simulink library "LiBatteryElements_lib"  (R2020b)
settings: Solver=VariableStepAuto  StartTime=0.0  StopTime=10.0  RelTol=1e-3
values from neighbouring files (symbols this model uses):
  A_an = 2.5e13    (= 25000000000000)    [main_cell.m]
  A_ca = 2.55e14    (= 255000000000000)    [main_cell.m]
  A_sei = 2.25e15    (= 2.25e+15)    [main_cell.m]
  capacity = 4.5    [Cell_1_RC_25.mat]    (also in Cell_43_RC_25.mat; parameters.mat = 10)
  E_an = 2.24e-19    [main_cell.m]
  E_ca = 2.64e-19    [main_cell.m]
  E_sei = 2.24e-19    [main_cell.m]
  h_an = 1714*1000    (= 1714000)    [main_cell.m]
  h_ca = 790*1000    (= 790000)    [main_cell.m]
  h_sei = 257*1000    (= 257000)    [main_cell.m]
  k_b = 1.3806e-23    [main_cell.m]
  m_an = 19.107/1000    (= 0.019107)    [main_cell.m]
  m_ca = 36.56/1000    (= 0.03656)    [main_cell.m]
  x_an_0 = 0.75    [main_cell.m]
  x_sei_0 = 0.15    [main_cell.m]
  z_0 = 0.033    [main_cell.m]
undefined symbols (not defined in the file or in its folder): gcbh, simscape, T_init
libraries: fl_lib x14, $bdroot x4, nesl_utility x4
settings Model: Creator=Vivian  LastModifiedBy=Vivian

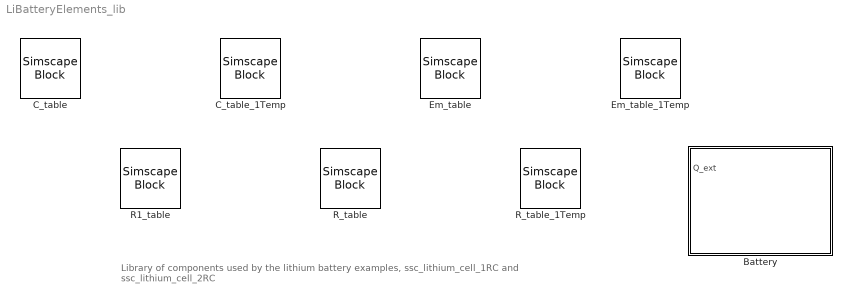
== system LiBatteryElements_lib ==
  note: Library of components used by the lithium battery examples, ssc_lithium_cell_1RC and ssc_lithium_cell_2RC
  Battery : Subsystem
  C_table : SimscapeBlock  DialogController=NetworkEngine.DynNeDlgSource  LoadFcn=simscape.compiler.sli.internal.callback('LoadFcn',gcbh);  SourceFile=LiBatteryElements.C_table  mask(C_table){ComponentPath=LiBatteryElements.C_table, ComponentVariants=["LiBatteryElements.C_table"], ComponentVariantNames=["C_table"], ClassName=C_table, SchemaVersion=1, C_Table=ones(5, 3), C_Table_unit=F, C_Table_conf=compiletime, SOC_Table=[0; .1; .5; .9; 1], SOC_Table_unit=1, SOC_Table_conf=compiletime, Temp_Table=[273.15, 293.15, 313.15], Temp_Table_unit=K, Temp_Table_conf=compiletime, v0=0, v0_unit=V, v0_conf=compiletime}
      mask prompts: C_Table "Matrix of capacitance values, C(SOC,T)"; SOC_Table "State of charge (SOC) breakpoints"; Temp_Table "Temperature (T) breakpoints"; v0 "Initial voltage across capacitor"
      mask help: Models a capacitor where the capacitance value (C) depends on an external physical signal inputs SOC and T. It is assumed that the capacitance value is slowly varying with time, and hence the equation i = C*dv/dt holds.
      mask init:
      | simscape.compiler.sli.internal.preinitmask(gcb);
      settings: CopyFcn=simscape.compiler.sli.internal.callback('CopyFcn',gcbh);  DeleteFcn=simscape.compiler.sli.internal.callback('DeleteFcn',gcbh);  ModelCloseFcn=simscape.compiler.sli.internal.callback('ModelCloseFcn',gcbh);  PreSaveFcn=simscape.compiler.sli.internal.callback('PreSaveFcn',gcbh);  PostSaveFcn=simscape.compiler.sli.internal.callback('PostSaveFcn',gcbh);  PreCopyFcn=simscape.compiler.sli.internal.callback('PreCopyFcn',gcbh);  PreDeleteFcn=simscape.compiler.sli.internal.callback('PreDeleteFcn',gcbh);  InternalSimscapePortConfiguration="{\"Bottom\":[],\"Left\":[{\"id\":\"p\",\"label\":\"+\",\"type\":\"foundation.electrical.electrical\"},{\"id\":\"T\",\"label\":\"T\",\"type\":\"input\"},{\"id\":\"SOC\",\"label\":\"SOC\",\"type\":\"input\"}],\"Right\":[{\"id\":\"n\",\"label\":\"-\",\"type\":\"foundation.electrical.electrical\"}],\"Top\":[]}"
      mask Help: web(nesl_help(gcbh))
      mask TypeOptions C_Table_unit: F | pF | nF | uF | mF
      mask TypeOptions C_Table_conf: compiletime | runtime
      mask TypeOptions SOC_Table_unit: 1
      mask TypeOptions SOC_Table_conf: compiletime | runtime
      mask TypeOptions Temp_Table_unit: K | degC | degF | degR | deltaK | deltadegC | deltadegF | deltadegR
      mask TypeOptions Temp_Table_conf: compiletime | runtime
      mask TypeOptions v0_unit: V | mV | kV
      mask TypeOptions v0_conf: compiletime | runtime
  C_table_1Temp : SimscapeBlock  DialogController=NetworkEngine.DynNeDlgSource  LoadFcn=simscape.compiler.sli.internal.callback('LoadFcn',gcbh);  SourceFile=LiBatteryElements.C_table_1Temp  mask(C_table_1Temp){ComponentPath=LiBatteryElements.C_table_1Temp, ComponentVariants=["LiBatteryElements.C_table_1Temp"], ComponentVariantNames=["C_table_1Temp"], ClassName=C_table_1Temp, SchemaVersion=1, C_Table=ones(5, 1), C_Table_unit=F, C_Table_conf=compiletime, SOC_Table=[0; .1; .5; .9; 1], SOC_Table_unit=1, SOC_Table_conf=compiletime, v0=0, v0_unit=V, v0_conf=compiletime}
      mask prompts: C_Table "Vector of capacitance values"; SOC_Table "Corresponding SOC breakpoints"; v0 "Initial voltage across capacitor"
      mask help: Models a capacitor where the capacitance value (C) depends on an external physical signal input SOC. It is assumed that the capacitance value is slowly varying with time, and hence the equation i = C*dv/dt holds.
      mask init:
      | simscape.compiler.sli.internal.preinitmask(gcb);
      settings: CopyFcn=simscape.compiler.sli.internal.callback('CopyFcn',gcbh);  DeleteFcn=simscape.compiler.sli.internal.callback('DeleteFcn',gcbh);  ModelCloseFcn=simscape.compiler.sli.internal.callback('ModelCloseFcn',gcbh);  PreSaveFcn=simscape.compiler.sli.internal.callback('PreSaveFcn',gcbh);  PostSaveFcn=simscape.compiler.sli.internal.callback('PostSaveFcn',gcbh);  PreCopyFcn=simscape.compiler.sli.internal.callback('PreCopyFcn',gcbh);  PreDeleteFcn=simscape.compiler.sli.internal.callback('PreDeleteFcn',gcbh);  InternalSimscapePortConfiguration="{\"Bottom\":[],\"Left\":[{\"id\":\"p\",\"label\":\"+\",\"type\":\"foundation.electrical.electrical\"},{\"id\":\"SOC\",\"label\":\"SOC\",\"type\":\"input\"}],\"Right\":[{\"id\":\"n\",\"label\":\"-\",\"type\":\"foundation.electrical.electrical\"}],\"Top\":[]}"
      mask Help: web(nesl_help(gcbh))
      mask TypeOptions C_Table_unit: F | pF | nF | uF | mF
      mask TypeOptions C_Table_conf: compiletime | runtime
      mask TypeOptions SOC_Table_unit: 1
      mask TypeOptions SOC_Table_conf: compiletime | runtime
      mask TypeOptions v0_unit: V | mV | kV
      mask TypeOptions v0_conf: compiletime | runtime
  Em_table : SimscapeBlock  DialogController=NetworkEngine.DynNeDlgSource  LoadFcn=simscape.compiler.sli.internal.callback('LoadFcn',gcbh);  SourceFile=LiBatteryElements.Em_table  mask(Em_table){ComponentPath=LiBatteryElements.Em_table, ComponentVariants=["LiBatteryElements.Em_table"], ComponentVariantNames=["Em_table"], ClassName=Em_table, SchemaVersion=1, C_Table=[29, 30, 31], C_Table_unit=hr*A, C_Table_conf=compiletime, Em_Table=3.8 * ones(5, 3), Em_Table_unit=V, Em_Table_conf=compiletime, SOC_Table=[0; .1; .5; .9; 1], SOC_Table_unit=1, SOC_Table_conf=compiletime, Temp_Table=[273.15, 293.15, 313.15], Temp_Table_unit=K, Temp_Table_conf=compiletime, Qinit=0, Qinit_unit=hr*A, Qinit_conf=compiletime}
      mask prompts: C_Table "Capacity values at specified temperature breakpoints"; Em_Table "Matrix of voltage values, Em(SOC,T)"; SOC_Table "State of charge (SOC) breakpoints"; Temp_Table "Temperature (T) breakpoints"; Qinit "Initial charge deficit"
      mask help: This block implements the cell's main branch voltage source, and determines values for capacity (C) and state of charge (SOC). The defining equations depend on cell temperature, T.
      mask init:
      | simscape.compiler.sli.internal.preinitmask(gcb);
      settings: CopyFcn=simscape.compiler.sli.internal.callback('CopyFcn',gcbh);  DeleteFcn=simscape.compiler.sli.internal.callback('DeleteFcn',gcbh);  ModelCloseFcn=simscape.compiler.sli.internal.callback('ModelCloseFcn',gcbh);  PreSaveFcn=simscape.compiler.sli.internal.callback('PreSaveFcn',gcbh);  PostSaveFcn=simscape.compiler.sli.internal.callback('PostSaveFcn',gcbh);  PreCopyFcn=simscape.compiler.sli.internal.callback('PreCopyFcn',gcbh);  PreDeleteFcn=simscape.compiler.sli.internal.callback('PreDeleteFcn',gcbh);  InternalSimscapePortConfiguration="{\"Bottom\":[],\"Left\":[{\"id\":\"p\",\"label\":\"+\",\"type\":\"foundation.electrical.electrical\"},{\"id\":\"C\",\"label\":\"C\",\"type\":\"output\"},{\"id\":\"SOC\",\"label\":\"SOC\",\"type\":\"output\"}],\"Right\":[{\"id\":\"n\",\"label\":\"-\",\"type\":\"foundation.electrical.electrical\"},{\"id\":\"T\",\"label\":\"T\",\"type\":\"input\"}],\"Top\":[]}"
      mask Help: web(nesl_help(gcbh))
      mask TypeOptions C_Table_unit: C | hr*A
      mask TypeOptions C_Table_conf: compiletime | runtime
      mask TypeOptions Em_Table_unit: V | mV | kV
      mask TypeOptions Em_Table_conf: compiletime | runtime
      mask TypeOptions SOC_Table_unit: 1
      mask TypeOptions SOC_Table_conf: compiletime | runtime
      mask TypeOptions Temp_Table_unit: K | degC | degF | degR | deltaK | deltadegC | deltadegF | deltadegR
      mask TypeOptions Temp_Table_conf: compiletime | runtime
      mask TypeOptions Qinit_unit: C | hr*A
      mask TypeOptions Qinit_conf: compiletime | runtime
  Em_table_1Temp : SimscapeBlock  DialogController=NetworkEngine.DynNeDlgSource  LoadFcn=simscape.compiler.sli.internal.callback('LoadFcn',gcbh);  SourceFile=LiBatteryElements.Em_table_1Temp  mask(Em_table_1Temp){ComponentPath=LiBatteryElements.Em_table_1Temp, ComponentVariants=["LiBatteryElements.Em_table_1Temp"], ComponentVariantNames=["Em_table_1Temp"], ClassName=Em_table_1Temp, SchemaVersion=1, Em_Table=3.8 * ones(5, 1), Em_Table_unit=V, Em_Table_conf=compiletime, SOC_Table=[0; .1; .5; .9; 1], SOC_Table_unit=1, SOC_Table_conf=compiletime, C=30, C_unit=hr*A, C_conf=compiletime, Qinit=0, Qinit_unit=hr*A, Qinit_conf=compiletime}
      mask prompts: Em_Table "Vector of voltage values, Em"; SOC_Table "Corresponding SOC breakpoints"; C "Capacity (scalar)"; Qinit "Initial charge deficit"
      mask help: This block implements the main branch voltage source, capacity, and state of charge (SOC). The defining equations are assumed not to depend on temperature.
      mask init:
      | simscape.compiler.sli.internal.preinitmask(gcb);
      settings: CopyFcn=simscape.compiler.sli.internal.callback('CopyFcn',gcbh);  DeleteFcn=simscape.compiler.sli.internal.callback('DeleteFcn',gcbh);  ModelCloseFcn=simscape.compiler.sli.internal.callback('ModelCloseFcn',gcbh);  PreSaveFcn=simscape.compiler.sli.internal.callback('PreSaveFcn',gcbh);  PostSaveFcn=simscape.compiler.sli.internal.callback('PostSaveFcn',gcbh);  PreCopyFcn=simscape.compiler.sli.internal.callback('PreCopyFcn',gcbh);  PreDeleteFcn=simscape.compiler.sli.internal.callback('PreDeleteFcn',gcbh);  InternalSimscapePortConfiguration="{\"Bottom\":[],\"Left\":[{\"id\":\"p\",\"label\":\"+\",\"type\":\"foundation.electrical.electrical\"},{\"id\":\"SOC\",\"label\":\"SOC\",\"type\":\"output\"}],\"Right\":[{\"id\":\"n\",\"label\":\"-\",\"type\":\"foundation.electrical.electrical\"}],\"Top\":[]}"
      mask Help: web(nesl_help(gcbh))
      mask TypeOptions Em_Table_unit: V | mV | kV
      mask TypeOptions Em_Table_conf: compiletime | runtime
      mask TypeOptions SOC_Table_unit: 1
      mask TypeOptions SOC_Table_conf: compiletime | runtime
      mask TypeOptions C_unit: C | hr*A
      mask TypeOptions C_conf: compiletime | runtime
      mask TypeOptions Qinit_unit: C | hr*A
      mask TypeOptions Qinit_conf: compiletime | runtime
  R1_table : SimscapeBlock  DialogController=NetworkEngine.DynNeDlgSource  LoadFcn=simscape.compiler.sli.internal.callback('LoadFcn',gcbh);  SourceFile=LiBatteryElements.R1_table  mask(R1_table){ComponentPath=LiBatteryElements.R1_table, ComponentVariants=["LiBatteryElements.R1_table"], ComponentVariantNames=["R1_table"], ClassName=R1_table, SchemaVersion=1, R_Table=1e-3 * ones(5, 3), R_Table_unit=Ohm, R_Table_conf=compiletime, SOC_Table=[0; .1; .5; .9; 1], SOC_Table_unit=1, SOC_Table_conf=compiletime, Temp_Table=[273.15, 293.15, 313.15], Temp_Table_unit=K, Temp_Table_conf=compiletime}
      mask prompts: R_Table "Matrix of resistance values, R(SOC,T)"; SOC_Table "State of charge (SOC) breakpoints"; Temp_Table "Temperature (T) breakpoints"
      mask help: Models a resistor where the resistance value (R) depends on an external physical signal inputs SOC and T.
      mask init:
      | simscape.compiler.sli.internal.preinitmask(gcb);
      settings: CopyFcn=simscape.compiler.sli.internal.callback('CopyFcn',gcbh);  DeleteFcn=simscape.compiler.sli.internal.callback('DeleteFcn',gcbh);  ModelCloseFcn=simscape.compiler.sli.internal.callback('ModelCloseFcn',gcbh);  PreSaveFcn=simscape.compiler.sli.internal.callback('PreSaveFcn',gcbh);  PostSaveFcn=simscape.compiler.sli.internal.callback('PostSaveFcn',gcbh);  PreCopyFcn=simscape.compiler.sli.internal.callback('PreCopyFcn',gcbh);  PreDeleteFcn=simscape.compiler.sli.internal.callback('PreDeleteFcn',gcbh);  InternalSimscapePortConfiguration="{\"Bottom\":[],\"Left\":[{\"id\":\"p\",\"label\":\"+\",\"type\":\"foundation.electrical.electrical\"},{\"id\":\"T\",\"label\":\"T\",\"type\":\"input\"},{\"id\":\"SOC\",\"label\":\"SOC\",\"type\":\"input\"}],\"Right\":[{\"id\":\"n\",\"label\":\"-\",\"type\":\"foundation.electrical.electrical\"},{\"id\":\"pow\",\"label\":\"POW\",\"type\":\"output\"}],\"Top\":[]}"
      mask Help: web(nesl_help(gcbh))
      mask TypeOptions R_Table_unit: Ohm | kOhm | MOhm | GOhm
      mask TypeOptions R_Table_conf: compiletime | runtime
      mask TypeOptions SOC_Table_unit: 1
      mask TypeOptions SOC_Table_conf: compiletime | runtime
      mask TypeOptions Temp_Table_unit: K | degC | degF | degR | deltaK | deltadegC | deltadegF | deltadegR
      mask TypeOptions Temp_Table_conf: compiletime | runtime
  R_table : SimscapeBlock  DialogController=NetworkEngine.DynNeDlgSource  LoadFcn=simscape.compiler.sli.internal.callback('LoadFcn',gcbh);  SourceFile=LiBatteryElements.R_table  mask(R_table){ComponentPath=LiBatteryElements.R_table, ComponentVariants=["LiBatteryElements.R_table"], ComponentVariantNames=["R_table"], ClassName=R_table, SchemaVersion=1, R_Table=1e-3 * ones(5, 3), R_Table_unit=Ohm, R_Table_conf=compiletime, SOC_Table=[0; .1; .5; .9; 1], SOC_Table_unit=1, SOC_Table_conf=compiletime, Temp_Table=[273.15, 293.15, 313.15], Temp_Table_unit=K, Temp_Table_conf=compiletime}
      mask prompts: R_Table "Matrix of resistance values, R(SOC,T)"; SOC_Table "State of charge (SOC) breakpoints"; Temp_Table "Temperature (T) breakpoints"
      mask help: Models a resistor where the resistance value (R) depends on an external physical signal inputs SOC and T.
      mask init:
      | simscape.compiler.sli.internal.preinitmask(gcb);
      settings: CopyFcn=simscape.compiler.sli.internal.callback('CopyFcn',gcbh);  DeleteFcn=simscape.compiler.sli.internal.callback('DeleteFcn',gcbh);  ModelCloseFcn=simscape.compiler.sli.internal.callback('ModelCloseFcn',gcbh);  PreSaveFcn=simscape.compiler.sli.internal.callback('PreSaveFcn',gcbh);  PostSaveFcn=simscape.compiler.sli.internal.callback('PostSaveFcn',gcbh);  PreCopyFcn=simscape.compiler.sli.internal.callback('PreCopyFcn',gcbh);  PreDeleteFcn=simscape.compiler.sli.internal.callback('PreDeleteFcn',gcbh);  InternalSimscapePortConfiguration="{\"Bottom\":[],\"Left\":[{\"id\":\"p\",\"label\":\"+\",\"type\":\"foundation.electrical.electrical\"},{\"id\":\"T\",\"label\":\"T\",\"type\":\"input\"},{\"id\":\"SOC\",\"label\":\"SOC\",\"type\":\"input\"}],\"Right\":[{\"id\":\"n\",\"label\":\"-\",\"type\":\"foundation.electrical.electrical\"},{\"id\":\"pow\",\"label\":\"POW\",\"type\":\"output\"}],\"Top\":[]}"
      mask Help: web(nesl_help(gcbh))
      mask TypeOptions R_Table_unit: Ohm | kOhm | MOhm | GOhm
      mask TypeOptions R_Table_conf: compiletime | runtime
      mask TypeOptions SOC_Table_unit: 1
      mask TypeOptions SOC_Table_conf: compiletime | runtime
      mask TypeOptions Temp_Table_unit: K | degC | degF | degR | deltaK | deltadegC | deltadegF | deltadegR
      mask TypeOptions Temp_Table_conf: compiletime | runtime
  R_table_1Temp : SimscapeBlock  DialogController=NetworkEngine.DynNeDlgSource  LoadFcn=simscape.compiler.sli.internal.callback('LoadFcn',gcbh);  SourceFile=LiBatteryElements.R_table_1Temp  mask(R_table_1Temp){ComponentPath=LiBatteryElements.R_table_1Temp, ComponentVariants=["LiBatteryElements.R_table_1Temp"], ComponentVariantNames=["R_table_1Temp"], ClassName=R_table_1Temp, SchemaVersion=1, R_Table=1e-3 * ones(5, 1), R_Table_unit=Ohm, R_Table_conf=compiletime, SOC_Table=[0; .1; .5; .9; 1], SOC_Table_unit=1, SOC_Table_conf=compiletime}
      mask prompts: R_Table "Vector of resistance values"; SOC_Table "Corresponding SOC breakpoints"
      mask help: Models a resistor where the resistance value (R) depends on an external physical signal input SOC.
      mask init:
      | simscape.compiler.sli.internal.preinitmask(gcb);
      settings: CopyFcn=simscape.compiler.sli.internal.callback('CopyFcn',gcbh);  DeleteFcn=simscape.compiler.sli.internal.callback('DeleteFcn',gcbh);  ModelCloseFcn=simscape.compiler.sli.internal.callback('ModelCloseFcn',gcbh);  PreSaveFcn=simscape.compiler.sli.internal.callback('PreSaveFcn',gcbh);  PostSaveFcn=simscape.compiler.sli.internal.callback('PostSaveFcn',gcbh);  PreCopyFcn=simscape.compiler.sli.internal.callback('PreCopyFcn',gcbh);  PreDeleteFcn=simscape.compiler.sli.internal.callback('PreDeleteFcn',gcbh);  InternalSimscapePortConfiguration="{\"Bottom\":[],\"Left\":[{\"id\":\"p\",\"label\":\"+\",\"type\":\"foundation.electrical.electrical\"},{\"id\":\"SOC\",\"label\":\"SOC\",\"type\":\"input\"}],\"Right\":[{\"id\":\"n\",\"label\":\"-\",\"type\":\"foundation.electrical.electrical\"}],\"Top\":[]}"
      mask Help: web(nesl_help(gcbh))
      mask TypeOptions R_Table_unit: Ohm | kOhm | MOhm | GOhm
      mask TypeOptions R_Table_conf: compiletime | runtime
      mask TypeOptions SOC_Table_unit: 1
      mask TypeOptions SOC_Table_conf: compiletime | runtime

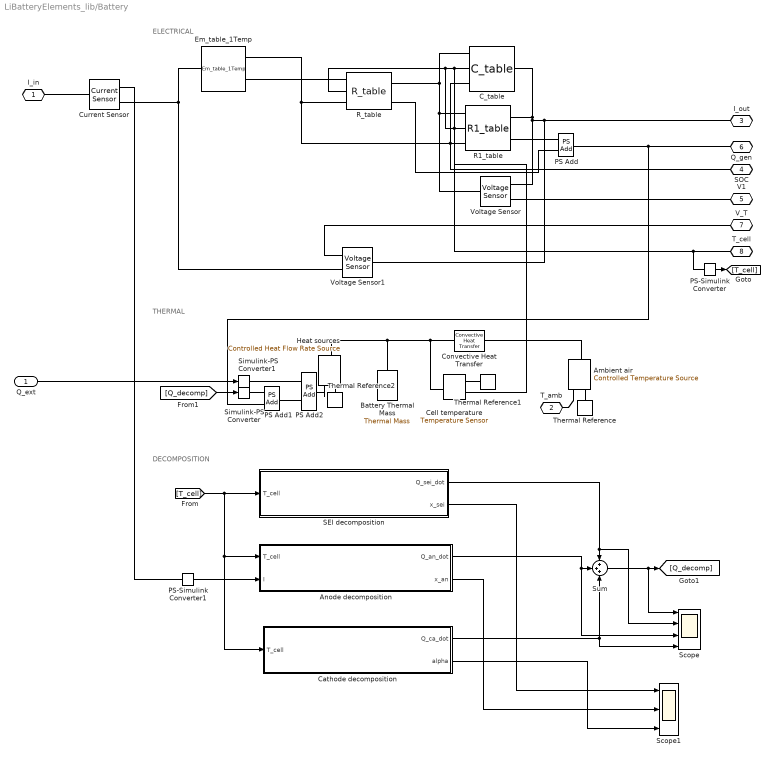
== system LiBatteryElements_lib/Battery ==
  note: ELECTRICAL
  note: THERMAL
  note: DECOMPOSITION
  Q_ext : Inport
  Ambient air : fl_lib/Thermal/Thermal Sources/Controlled Temperature Source
  Anode decomposition : Subsystem
  Battery Thermal Mass : fl_lib/Thermal/Thermal Elements/Thermal Mass  mass=cell_mass kg  sp_heat=cell_Cp_heat J/kg/K  T_specify=on  T_priority=High  T=T_init K  T_nominal_specify=off  T_nominal_unit=K  T_nominal_value=1  Q_specify=on  Q_priority=None  Q=0 W  Q_nominal_specify=off  Q_nominal_unit=W  Q_nominal_value=1
  C_table : $bdroot/C_table  C_Table=ones(5, 3) F  SOC_Table=[0; .1; .5; .9; 1]  Temp_Table=[273.15, 293.15, 313.15] K  v0=0 V
      settings: InternalSimscapePortConfiguration="{\"Bottom\":[],\"Left\":[{\"id\":\"p\",\"label\":\"+\",\"type\":\"foundation.electrical.electrical\"},{\"id\":\"T\",\"label\":\"T\",\"type\":\"input\"},{\"id\":\"SOC\",\"label\":\"SOC\",\"type\":\"input\"}],\"Right\":[{\"id\":\"n\",\"label\":\"-\",\"type\":\"foundation.electrical.electrical\"}],\"Top\":[]}"
  Cathode decomposition : Subsystem
  Cell temperature : fl_lib/Thermal/Thermal Sensors/Temperature Sensor
  Convective Heat Transfer : fl_lib/Thermal/Thermal Elements/Convective Heat Transfer  area=cell_area m^2  heat_tr_coeff=h_conv W/(m^2 * K)  T_specify=off  T_priority=None  T=0 K  T_nominal_specify=off  T_nominal_unit=K  T_nominal_value=1  Q_specify=off  Q_priority=None  Q=0 W  Q_nominal_specify=off  Q_nominal_unit=W  Q_nominal_value=1
  Current Sensor : fl_lib/Electrical/Electrical Sensors/Current Sensor
  Em_table_1Temp : $bdroot/Em_table_1Temp  Em_Table=3.8 * ones(5, 1) V  SOC_Table=[0; .1; .5; .9; 1]  C=30 hr*A  Qinit=0 hr*A
      settings: InternalSimscapePortConfiguration="{\"Bottom\":[],\"Left\":[{\"id\":\"p\",\"label\":\"+\",\"type\":\"foundation.electrical.electrical\"},{\"id\":\"SOC\",\"label\":\"SOC\",\"type\":\"output\"}],\"Right\":[{\"id\":\"n\",\"label\":\"-\",\"type\":\"foundation.electrical.electrical\"}],\"Top\":[]}"
  Heat sources : fl_lib/Thermal/Thermal Sources/Controlled Heat Flow Rate Source
  PS Add : fl_lib/Physical Signals/Functions/PS Add
  PS Add1 : fl_lib/Physical Signals/Functions/PS Add
  PS Add2 : fl_lib/Physical Signals/Functions/PS Add
  PS-Simulink Converter : nesl_utility/PS-Simulink Converter  PhysicalDomain=network_engine_domain  SubClassName=ps_output  LeftPortType=input  RightPortType=output  PseudoPeriodic=off  Frequencies=[]  Unit=inherit  AffineConversion=off
  PS-Simulink Converter1 : nesl_utility/PS-Simulink Converter  PhysicalDomain=network_engine_domain  SubClassName=ps_output  LeftPortType=input  RightPortType=output  PseudoPeriodic=off  Frequencies=[]  Unit=inherit  AffineConversion=off
  R1_table : $bdroot/R1_table  R_Table=1e-3 * ones(5, 3) Ohm  SOC_Table=[0; .1; .5; .9; 1]  Temp_Table=[273.15, 293.15, 313.15] K
      settings: InternalSimscapePortConfiguration="{\"Bottom\":[],\"Left\":[{\"id\":\"p\",\"label\":\"+\",\"type\":\"foundation.electrical.electrical\"},{\"id\":\"T\",\"label\":\"T\",\"type\":\"input\"},{\"id\":\"SOC\",\"label\":\"SOC\",\"type\":\"input\"}],\"Right\":[{\"id\":\"n\",\"label\":\"-\",\"type\":\"foundation.electrical.electrical\"},{\"id\":\"pow\",\"label\":\"POW\",\"type\":\"output\"}],\"Top\":[]}"
  R_table : $bdroot/R_table  R_Table=1e-3 * ones(5, 3) Ohm  SOC_Table=[0; .1; .5; .9; 1]  Temp_Table=[273.15, 293.15, 313.15] K
      settings: InternalSimscapePortConfiguration="{\"Bottom\":[],\"Left\":[{\"id\":\"p\",\"label\":\"+\",\"type\":\"foundation.electrical.electrical\"},{\"id\":\"T\",\"label\":\"T\",\"type\":\"input\"},{\"id\":\"SOC\",\"label\":\"SOC\",\"type\":\"input\"}],\"Right\":[{\"id\":\"n\",\"label\":\"-\",\"type\":\"foundation.electrical.electrical\"},{\"id\":\"pow\",\"label\":\"POW\",\"type\":\"output\"}],\"Top\":[]}"
  SEI decomposition : Subsystem
  Scope : Scope  NumInputPorts=4
  Scope1 : Scope  NumInputPorts=3
  Simulink-PS Converter : nesl_utility/Simulink-PS Converter  PhysicalDomain=network_engine_domain  SubClassName=ps_input  LeftPortType=input  RightPortType=output  PseudoPeriodic=off  Frequencies=[]  NoiseDistribution=none  NoiseParameters=[]  Unit=W  AffineConversion=off  FilteringAndDerivatives=provide  SimscapeFilterOrder=1  InputFilterTimeConstant=0.001  UdotUserProvided=0
  Simulink-PS Converter1 : nesl_utility/Simulink-PS Converter  PhysicalDomain=network_engine_domain  SubClassName=ps_input  LeftPortType=input  RightPortType=output  PseudoPeriodic=off  Frequencies=[]  NoiseDistribution=none  NoiseParameters=[]  Unit=W  AffineConversion=off  FilteringAndDerivatives=provide  SimscapeFilterOrder=1  InputFilterTimeConstant=0.001  UdotUserProvided=0
  Sum : Sum  Inputs=+++
  Thermal Reference : fl_lib/Thermal/Thermal Elements/Thermal Reference
  Thermal Reference1 : fl_lib/Thermal/Thermal Elements/Thermal Reference
  Thermal Reference2 : fl_lib/Thermal/Thermal Elements/Thermal Reference
  Voltage Sensor : fl_lib/Electrical/Electrical Sensors/Voltage Sensor
  Voltage Sensor1 : fl_lib/Electrical/Electrical Sensors/Voltage Sensor
  I_in : PMIOPort  Side=Left
  T_amb : PMIOPort  Port=2  Side=Left
  I_out : PMIOPort  Port=3  Side=Right
  SOC : PMIOPort  Port=4  Side=Right
  V1 : PMIOPort  Port=5  Side=Right
  Q_gen : PMIOPort  Port=6  Side=Right
  V_T : PMIOPort  Port=7  Side=Right
  T_cell : PMIOPort  Port=8  Side=Right
  wires:
  PS-Simulink Converter1/1 -> Anode decomposition/2(I)
  Q_ext/1 -> Simulink-PS Converter1/1
  Cathode decomposition/2(alpha) -> Scope1/3
  Anode decomposition/2(x_an) -> Scope1/2
  SEI decomposition/2(x_sei) -> Scope1/1
  Cathode decomposition/1(Q_ca_dot) -> Sum/3, Scope/4
  SEI decomposition/1(Q_sei_dot) -> Sum/1, Scope/2
  Anode decomposition/1(Q_an_dot) -> Sum/2, Scope/3
  Sum/1 -> [Q_decomp], Scope/1
  [T_cell] -> SEI decomposition/1(T_cell), Anode decomposition/1(T_cell), Cathode decomposition/1(T_cell)
  [Q_decomp] -> Simulink-PS Converter/1
  PS-Simulink Converter/1 -> [T_cell]
  connections:
  Current Sensor/RConn1 -- PS-Simulink Converter1/LConn1
  Current Sensor/LConn1 -- I_in/RConn1
  Simulink-PS Converter1/RConn1 -- PS Add2/LConn1
  Heat sources/RConn1 -- PS Add2/RConn1
  PS Add2/LConn2 -- PS Add1/RConn1
  PS Add1/LConn1 -- Simulink-PS Converter/RConn1
  Thermal Reference2/LConn1 -- Heat sources/RConn2
  PS-Simulink Converter/LConn1 -- Cell temperature/RConn2 -- C_table/LConn2 -- R_table/LConn2 -- R1_table/LConn2 -- T_cell/RConn1
  Thermal Reference1/LConn1 -- Cell temperature/RConn1
  Thermal Reference/LConn1 -- Ambient air/RConn2
  Ambient air/RConn1 -- T_amb/RConn1
  Convective Heat Transfer/RConn1 -- Ambient air/LConn1
  Battery Thermal Mass/LConn1 -- Heat sources/LConn1 -- Convective Heat Transfer/LConn1 -- Cell temperature/LConn1
  Voltage Sensor/LConn1 -- R1_table/LConn1 -- C_table/LConn1 -- R_table/RConn1
  Voltage Sensor/RConn2 -- C_table/RConn1 -- R1_table/RConn1 -- Voltage Sensor1/LConn1 -- I_out/RConn1
  R_table/LConn1 -- Em_table_1Temp/LConn1
  PS Add1/LConn2 -- Q_gen/RConn1 -- PS Add/RConn1
  Current Sensor/RConn2 -- Em_table_1Temp/RConn1 -- Voltage Sensor1/RConn2
  SOC/RConn1 -- C_table/LConn3 -- R1_table/LConn3 -- Em_table_1Temp/LConn2 -- R_table/LConn3
  R1_table/RConn2 -- PS Add/LConn1
  Voltage Sensor1/RConn1 -- V_T/RConn1
  Voltage Sensor/RConn1 -- V1/RConn1
  R_table/RConn2 -- PS Add/LConn2

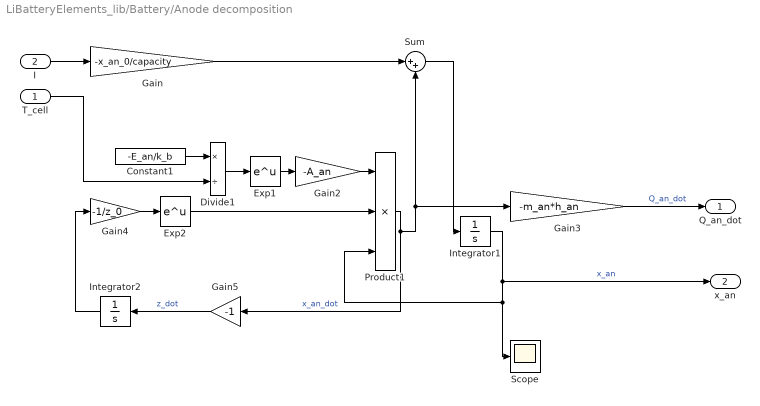
== system LiBatteryElements_lib/Battery/Anode decomposition ==
  T_cell : Inport
  I : Inport  Port=2
  Constant1 : Constant  Value=-E_an/k_b
  Divide1 : Product  Inputs=*/
  Exp1 : Math  SaturateOnIntegerOverflow=on
  Exp2 : Math  SaturateOnIntegerOverflow=on
  Gain : Gain  Gain=-x_an_0/capacity
  Gain2 : Gain  Gain=-A_an
  Gain3 : Gain  Gain=-m_an*h_an
  Gain4 : Gain  Gain=-1/z_0
  Gain5 : Gain  Gain=-1
  Integrator1 : Integrator  InitialCondition=x_an_0  LimitOutput=on  UpperSaturationLimit=x_an_0  LowerSaturationLimit=0
  Integrator2 : Integrator  InitialCondition=z_0  LimitOutput=on  LowerSaturationLimit=0
  Product1 : Product  Inputs=3
  Scope : Scope
  Sum : Sum  Inputs=|++
  Q_an_dot : Outport
  x_an : Outport  Port=2
  wires:
  Sum/1 -> Integrator1/1
  Gain/1 -> Sum/1
  I/1 -> Gain/1
  T_cell/1 -> Divide1/2
  Gain3/1 -> Q_an_dot/1  "Q_an_dot"
  Exp2/1 -> Product1/2
  Constant1/1 -> Divide1/1
  Gain4/1 -> Exp2/1
  Integrator1/1 -> x_an/1, Product1/3, Scope/1  "x_an"
  Exp1/1 -> Gain2/1
  Integrator2/1 -> Gain4/1
  Divide1/1 -> Exp1/1
  Gain5/1 -> Integrator2/1  "z_dot"
  Product1/1 -> Gain3/1, Sum/2, Gain5/1  "x_an_dot"
  Gain2/1 -> Product1/1

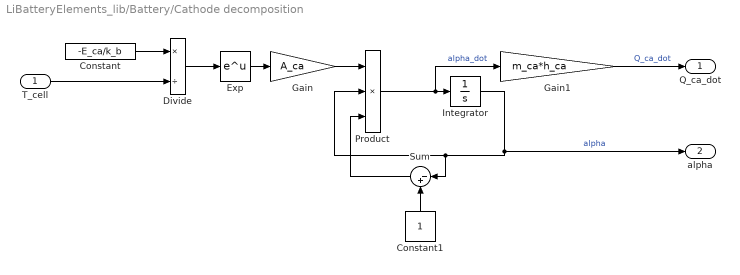
== system LiBatteryElements_lib/Battery/Cathode decomposition ==
  T_cell : Inport
  Constant : Constant  Value=-E_ca/k_b
  Constant1 : Constant
  Divide : Product  Inputs=*/
  Exp : Math  SaturateOnIntegerOverflow=on
  Gain : Gain  Gain=A_ca
  Gain1 : Gain  Gain=m_ca*h_ca
  Integrator : Integrator  InitialCondition=x_sei_0  LimitOutput=on  UpperSaturationLimit=x_sei_0  LowerSaturationLimit=0
  Product : Product  Inputs=3
  Sum : Sum  Inputs=|-+
  Q_ca_dot : Outport
  alpha : Outport  Port=2
  wires:
  Sum/1 -> Product/3
  Constant1/1 -> Sum/2
  Exp/1 -> Gain/1
  Divide/1 -> Exp/1
  T_cell/1 -> Divide/2
  Gain/1 -> Product/1
  Integrator/1 -> alpha/1, Product/2, Sum/1  "alpha"
  Gain1/1 -> Q_ca_dot/1  "Q_ca_dot"
  Product/1 -> Integrator/1, Gain1/1  "alpha_dot"
  Constant/1 -> Divide/1

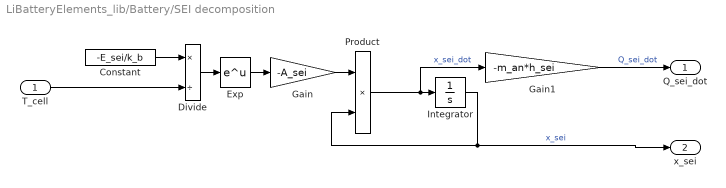
== system LiBatteryElements_lib/Battery/SEI decomposition ==
  T_cell : Inport
  Constant : Constant  Value=-E_sei/k_b
  Divide : Product  Inputs=*/
  Exp : Math  SaturateOnIntegerOverflow=on
  Gain : Gain  Gain=-A_sei
  Gain1 : Gain  Gain=-m_an*h_sei
  Integrator : Integrator  InitialCondition=x_sei_0  LimitOutput=on  UpperSaturationLimit=x_sei_0  LowerSaturationLimit=0
  Product : Product
  Q_sei_dot : Outport
  x_sei : Outport  Port=2
  wires:
  Exp/1 -> Gain/1
  Divide/1 -> Exp/1
  T_cell/1 -> Divide/2
  Gain/1 -> Product/1
  Integrator/1 -> Product/2, x_sei/1  "x_sei"
  Gain1/1 -> Q_sei_dot/1  "Q_sei_dot"
  Product/1 -> Integrator/1, Gain1/1  "x_sei_dot"
  Constant/1 -> Divide/1
